simulink model "SIMULINK_INVERSE_IDENTIFICATION_SANTIAGO_GARCIA"  (R2020a)
settings: Solver=FixedStepAuto  StartTime=0.0  StopTime=200  FixedStep=0.001  RelTol=1e-2
libraries: simulink x1
settings Model: Creator=elkin  LastModifiedBy=USUARIO

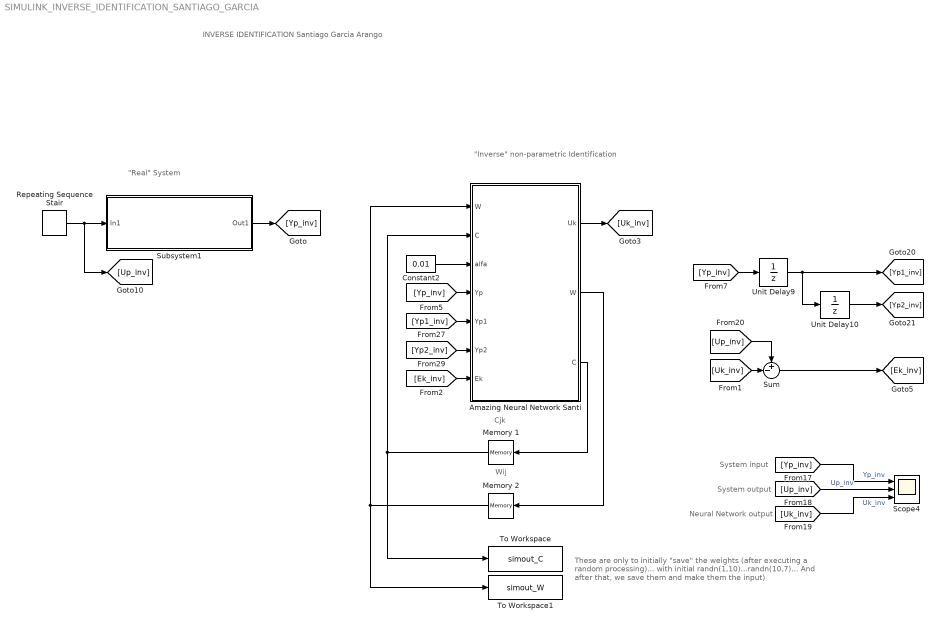
== system SIMULINK_INVERSE_IDENTIFICATION_SANTIAGO_GARCIA ==
  note: These are only to initially "save" the weights (after executing a random processing)... with initial randn(1,10)...randn(10,7)...
      | And after that,  we save them and make them the input)
  note: "Real" System
  note: INVERSE IDENTIFICATION
      | Santiago Garcia Arango
  note: "Inverse" non-parametric Identification
  note: Cjk
  note: Wij
  note: System input
  note: System output
  note: Neural Network output
  " Memory 2" : Memory  InitialCondition=randn(10,3)
  Amazing Neural Network Santi : MATLAB Function  TreatAsAtomicUnit=on
  Constant2 : Constant  Value=0.01
  Memory 1 : Memory  InitialCondition=randn(1,10)
  Repeating Sequence Stair : simulink/Sources/Repeating Sequence Stair  OutValues=[0 0.2 0 0.3 0.5 0.4 1].'  tsamp=20  OutMin=[]  OutMax=[]  OutDataTypeStr=double  OutputDataTypeScalingMode=double  OutDataType=fixdt(0,8)  ConRadixGroup=Best Precision: Vector-wise  OutScaling=2^-12
  Scope4 : Scope  NumInputPorts=3
  Subsystem1 : Subsystem
  Sum : Sum  Inputs=+-|
  To Workspace : ToWorkspace  VariableName=simout_C  SaveFormat=Timeseries  SampleTime=-1
  To Workspace1 : ToWorkspace  VariableName=simout_W  SaveFormat=Timeseries  SampleTime=-1
  Unit Delay10 : UnitDelay  SampleTime=-1  HasFrameUpgradeWarning=on
  Unit Delay9 : UnitDelay  SampleTime=-1  HasFrameUpgradeWarning=on
  wires:
  [Yp1_inv] -> Amazing Neural Network Santi/5(Yp1)
  Amazing Neural Network Santi/2(W) -> " Memory 2"/1
  [Yp2_inv] -> Amazing Neural Network Santi/6(Yp2)
  " Memory 2"/1 -> To Workspace1/1, Amazing Neural Network Santi/1("W ")
  Amazing Neural Network Santi/3(C) -> Memory 1/1
  [Yp_inv] -> Amazing Neural Network Santi/4(Yp)
  Constant2/1 -> Amazing Neural Network Santi/3(alfa)
  Memory 1/1 -> To Workspace/1, Amazing Neural Network Santi/2("C ")
  Amazing Neural Network Santi/1(Uk) -> [Uk_inv]
  [Yp_inv] -> Unit Delay9/1
  Unit Delay9/1 -> [Yp1_inv], Unit Delay10/1
  Unit Delay10/1 -> [Yp2_inv]
  Subsystem1/1(Out1) -> [Yp_inv]
  Repeating Sequence Stair/1 -> [Up_inv], Subsystem1/1(In1)
  [Up_inv] -> Scope4/2  "Up_inv"
  [Uk_inv] -> Scope4/3  "Uk_inv"
  [Yp_inv] -> Scope4/1  "Yp_inv"
  [Up_inv] -> Sum/1
  Sum/1 -> [Ek_inv]
  [Uk_inv] -> Sum/2
  [Ek_inv] -> Amazing Neural Network Santi/7(Ek)

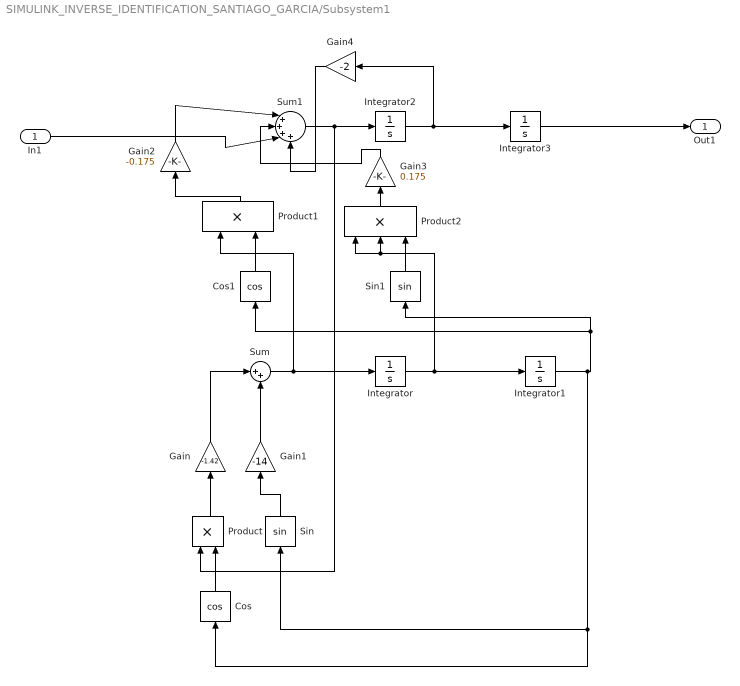
== system SIMULINK_INVERSE_IDENTIFICATION_SANTIAGO_GARCIA/Subsystem1 ==
  In1 : Inport
  Cos : Trigonometry  Operator=cos
  Cos1 : Trigonometry  Operator=cos
  Gain : Gain  Gain=-1.42
  Gain1 : Gain  Gain=-14
  Gain2 : Gain  Gain=-0.175
  Gain3 : Gain  Gain=0.175
  Gain4 : Gain  Gain=-2
  Integrator{,1..3} (4 alike) : Integrator
  Product : Product
  Product1 : Product
  Product2 : Product  Inputs=3
  Sin : Trigonometry
  Sin1 : Trigonometry
  Sum : Sum  Inputs=|++
  Sum1 : Sum  Inputs=|++++
  Out1 : Outport  VectorParamsAs1DForOutWhenUnconnected=off
  wires:
  Product2/1 -> Gain3/1
  Integrator3/1 -> Out1/1
  Sum/1 -> Integrator/1, Product1/1
  Integrator/1 -> Integrator1/1, Product2/1, Product2/2
  Integrator1/1 -> Sin/1, Cos/1, Cos1/1, Sin1/1
  Integrator2/1 -> Gain4/1, Integrator3/1
  Cos/1 -> Product/2
  Gain4/1 -> Sum1/4
  Sum1/1 -> Product/1, Integrator2/1
  Product1/1 -> Gain2/1
  Sin1/1 -> Product2/3
  In1/1 -> Sum1/3
  Gain1/1 -> Sum/2
  Gain/1 -> Sum/1
  Product/1 -> Gain/1
  Gain3/1 -> Sum1/2
  Sin/1 -> Gain1/1
  Gain2/1 -> Sum1/1
  Cos1/1 -> Product1/2

== matlab function SIMULINK_INVERSE_IDENTIFICATION_SANTIAGO_GARCIA/Amazing Neural Network Santi ==
  data: W input; Uk output; C input; alfa input; Yp input; Yp1 input; Yp2 input; W output; C output; Ek input
% NEURAL NETWORK FOR SIMULINK "REAL-TIME" PROCESSING BASED ON SIGNALS
% Santiago Garcia Arango
% ------------------------------------------------------------------------
% FEEDFORWARDMADALINE. Train or Test a simple neural network.
%   alfa: Learning rate constant (1 x 1)
%   W: vector of the initial Weights. size (1 x ne)
%   C: matrix of the initial hidden layers weights. size (ns x no+1)
%   REMARK: This processing is based on an "Inverse Identification"
% ------------------------------------------------------------------------

function [Uk, W, C] = fcn(W, C, alfa, Yp, Yp1, Yp2, Ek)

activation_function_1 = "tanh";
activation_function_2 = "none";

X = [Yp Yp1 Yp2]; % Create "entries" vector
Aj = W*X'; % Add hidden layer

if (activation_function_1 == "tanh")
    H = tanh(Aj);
end

Ak = C'*H; % Add output layer

if (activation_function_2 == "none")
    Uk = Ak;
end

C = C+alfa*Ek*H; % Update weights of C

if (activation_function_1 == "tanh")
    H2 = sech(Aj).^2;
end

W = W+alfa*Ek*(C.*H2)*X; % Update weights of W

end
